simulink model "desktop_subscribe"  (R2020a)
settings: Solver=FixedStepAuto  StartTime=0.0  StopTime=inf  RelTol=1e-3  EnableMultiTasking=on
PreLoadFcn:
  | Ts = 0.01;
model workspace (MAT data in the model file):
  SL_ROS_VariableLengthArrays_MaxSizes.CommonInfo.ArrayTruncateAction = 'EmitWarning'
  SL_ROS_VariableLengthArrays_MaxSizes.MsgTypeMap = containers.Map
  SL_ROS_VariableLengthArrays_MaxSizes.MsgTypeMap.serialization.keys = {'sensor_msgs/Image'}
  SL_ROS_VariableLengthArrays_MaxSizes.MsgTypeMap.serialization.values{1}(1).PropertyName = 'Data'
  SL_ROS_VariableLengthArrays_MaxSizes.MsgTypeMap.serialization.values{1}(1).DataType = 'uint8'
  SL_ROS_VariableLengthArrays_MaxSizes.MsgTypeMap.serialization.values{1}(1).MaxLength = 57600
  SL_ROS_VariableLengthArrays_MaxSizes.MsgTypeMap.serialization.values{1}(2).PropertyName = 'Encoding'
  SL_ROS_VariableLengthArrays_MaxSizes.MsgTypeMap.serialization.values{1}(2).DataType = 'uint8'
  SL_ROS_VariableLengthArrays_MaxSizes.MsgTypeMap.serialization.values{1}(2).MaxLength = 5
  SL_ROS_VariableLengthArrays_MaxSizes.MsgTypeMap.serialization.uniformity = 0
  SL_ROS_VariableLengthArrays_MaxSizes.MsgTypeMap.serialization.keyType = 'char'
  SL_ROS_VariableLengthArrays_MaxSizes.MsgTypeMap.serialization.valueType = 'any'
libraries: robotlib x2
settings Model: SimulationMode=external  Creator=The MathWorks, Inc.  LastModifiedBy=mmordeka
settings DataIOCC: SaveFormat=Array  ReturnWorkspaceOutputs=off
settings OptimizationCC: EnhancedBackFolding=on  PassReuseOutputArgsAs=Individual arguments  ZeroExternalMemoryAtStartup=off  ZeroInternalMemoryAtStartup=off  MaxStackSize=64  OptimizeBlockOrder=speed  DifferentSizesBufferReuse=on  OptimizationCustomize=off  EfficientTunableParamExpr=on
settings DebuggingCC: SolverPrmCheckMsg=warning  ParameterTunabilityLossMsg=error  AllowSymbolicDim=off  SFUnexpectedBacktrackingDiag=warning  SFNoUnconditionalDefaultTransitionDiag=warning  ArithmeticOperatorsInVariantConditions=warning
settings HardwareCC: ProdBitPerPointer=32  ProdBitPerSizeT=32  ProdBitPerPtrDiffT=32  ProdLargestAtomicInteger=Long  ProdLargestAtomicFloat=Double  ProdWordSize=32  ProdHWDeviceType=ARM Compatible->ARM Cortex
settings ModelReferenceCC: PropagateSignalLabelsOutOfModel=off
settings SFSimCC: SimUseLocalCustomCode=off  CustomCodeUndefinedFunction=UseInterfaceOnly
settings RTWCC: SystemTargetFile=ert.tlc  HardwareBoard=Raspberry Pi - Robot Operating System (ROS)  TemplateMakefile=ert_default_tmf  GenerateReport=on  RTWUseLocalCustomCode=off  Toolchain=Catkin  IncludeHyperlinkInReport=on  LaunchReport=on  TargetLang=C++  GenerateTraceInfo=on  GenerateTraceReport=on  GenerateTraceReportSl=on  GenerateTraceReportSf=on  GenerateTraceReportEml=on
settings CodeAppCC: ForceParamTrailComments=on  IgnoreCustomStorageClasses=off  OperatorAnnotations=on  SimulinkDataObjDesc=on  SFDataObjDesc=on  InsertBlockDesc=on
settings ERTTargetCC: ExtMode=on
settings ConfigComp: CovMetricSettings=dw  CovHtmlReporting=on  CovSaveCumulativeToWorkspaceVar=on  CovSaveSingleToWorkspaceVar=on  CovExternalEMLEnable=off  CovSFcnEnable=off

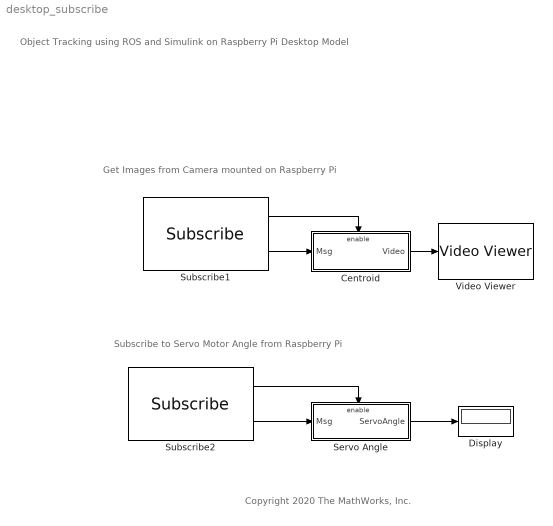
== system desktop_subscribe ==
  note: Copyright 2020 The MathWorks, Inc.
  note: Subscribe to Servo Motor Angle from Raspberry Pi
  note: Get Images from Camera mounted on Raspberry Pi
  note: Object Tracking using ROS and Simulink on Raspberry Pi
      | Desktop Model
  Centroid : Subsystem
  Display : Display
  Servo Angle : Subsystem
  Subscribe1 : robotlib/Subscribe  topicSource=Specify your own  topic=/camera  messageType=sensor_msgs/Image  sampleTime=Ts  messageQueueLength=51
  Subscribe2 : robotlib/Subscribe  topicSource=Specify your own  topic=/servo_angle  messageType=std_msgs/UInt8  sampleTime=Ts  messageQueueLength=51
  Video Viewer : VideoViewer  FigPos=[2041 741 418 304]
  wires:
  Subscribe1/1 -> Centroid/Enable
  Subscribe1/2 -> Centroid/1(Msg)
  Servo Angle/1(ServoAngle) -> Display/1
  Subscribe2/1 -> Servo Angle/Enable
  Subscribe2/2 -> Servo Angle/1(Msg)
  Centroid/1(Video) -> Video Viewer/1

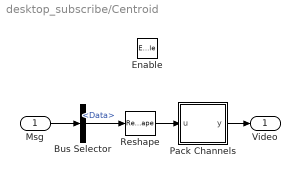
== system desktop_subscribe/Centroid ==
  Msg : Inport
  Enable : EnablePort
  Bus Selector : BusSelector  OutputSignals=Data
  Pack Channels : MATLAB Function  TreatAsAtomicUnit=on
  Reshape : Reshape  OutputDimensionality=Customize  OutputDimensions=[160 120 3]
  Video : Outport
  wires:
  Msg/1 -> Bus Selector/1
  Bus Selector/1 -> Reshape/1  "<Data>"
  Reshape/1 -> Pack Channels/1(u)
  Pack Channels/1(y) -> Video/1

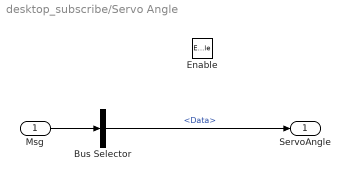
== system desktop_subscribe/Servo Angle ==
  Msg : Inport
  Enable : EnablePort
  Bus Selector : BusSelector  OutputSignals=Data
  ServoAngle : Outport
  wires:
  Bus Selector/1 -> ServoAngle/1  "<Data>"
  Msg/1 -> Bus Selector/1

== matlab function desktop_subscribe/Centroid/Pack Channels ==
  data: u input; y output
function y = fcn(u)

R = u(:,:,1)';
G = u(:,:,2)';
B = u(:,:,3)';

y = cat(3,R,G,B);
